simulink model "signal_builder"  (R2019b)
settings: Solver=VariableStepAuto  StartTime=0.0  StopTime=8760  RelTol=1e-3
undefined symbols (not defined in the file or in its folder): sigbuilder_block
settings Model: Creator=HP  LastModifiedBy=HP

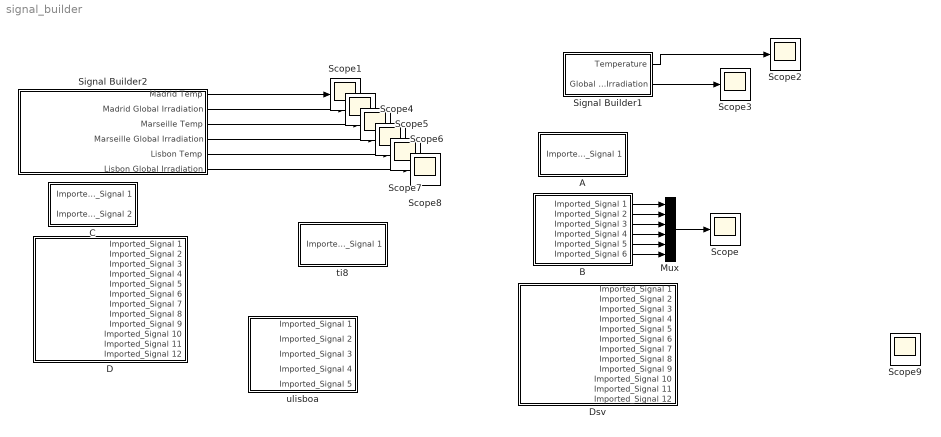
== system signal_builder ==
  A : Subsystem  Tag=STV Subsys  LoadFcn=sigbuilder_block('load');  StartFcn=sigbuilder_block('start');  StopFcn=sigbuilder_block('stop');  ClipboardFcn=sigbuilder_block('clipboard');  mask(Sigbuilder block){tuvar=[0:10]}
      mask help: Simulink:masks:SigbuilderBlock_MD
      mask init:
      | if ~strcmp(get_param(bdroot(gcbh),'SimulationStatus'),'stopped') tuvar = sigbuilder_block('maskInit'); end
      settings: CopyFcn=sigbuilder_block('copy');  DeleteFcn=sigbuilder_block('delete');  ModelCloseFcn=sigbuilder_block('modelClose');  PreSaveFcn=sigbuilder_block('preSave');  PauseFcn=sigbuilder_block('pause');  ContinueFcn=sigbuilder_block('continue');  NameChangeFcn=sigbuilder_block('namechange');  OpenFcn=sigbuilder_block('open',[437.6 153 550.4 359.25 ]);  CloseFcn=sigbuilder_block('close');
      mask Display: plot(0, 0, 100, 100,[2, 2, 32, 32, 2], [68, 8, 8, 68, 68],[32, 2], [38, 38], [32, 19, 2],[53, 60, 44], [32, 17, 17, 2],[16, 16, 31, 31]);txt = getActiveGroup(gcbh);text(2, 100, txt,'verticalAlignment', 'top');
  B : Subsystem  Tag=STV Subsys  LoadFcn=sigbuilder_block('load');  StartFcn=sigbuilder_block('start');  StopFcn=sigbuilder_block('stop');  ClipboardFcn=sigbuilder_block('clipboard');  mask(Sigbuilder block){tuvar=[0:10]}
      mask help: Simulink:masks:SigbuilderBlock_MD
      mask init:
      | if ~strcmp(get_param(bdroot(gcbh),'SimulationStatus'),'stopped') tuvar = sigbuilder_block('maskInit'); end
      settings: CopyFcn=sigbuilder_block('copy');  DeleteFcn=sigbuilder_block('delete');  ModelCloseFcn=sigbuilder_block('modelClose');  PreSaveFcn=sigbuilder_block('preSave');  PauseFcn=sigbuilder_block('pause');  ContinueFcn=sigbuilder_block('continue');  NameChangeFcn=sigbuilder_block('namechange');  OpenFcn=sigbuilder_block('open',[0 0 762.75 233.25 ]);  CloseFcn=sigbuilder_block('close');
      mask Display: plot(0, 0, 100, 100,[2, 2, 32, 32, 2], [68, 8, 8, 68, 68],[32, 2], [38, 38], [32, 19, 2],[53, 60, 44], [32, 17, 17, 2],[16, 16, 31, 31]);txt = getActiveGroup(gcbh);text(2, 100, txt,'verticalAlignment', 'top');
  C : Subsystem  Tag=STV Subsys  LoadFcn=sigbuilder_block('load');  StartFcn=sigbuilder_block('start');  StopFcn=sigbuilder_block('stop');  ClipboardFcn=sigbuilder_block('clipboard');  mask(Sigbuilder block){tuvar=[0:10]}
      mask help: Simulink:masks:SigbuilderBlock_MD
      mask init:
      | if ~strcmp(get_param(bdroot(gcbh),'SimulationStatus'),'stopped') tuvar = sigbuilder_block('maskInit'); end
      settings: CopyFcn=sigbuilder_block('copy');  DeleteFcn=sigbuilder_block('delete');  ModelCloseFcn=sigbuilder_block('modelClose');  PreSaveFcn=sigbuilder_block('preSave');  PauseFcn=sigbuilder_block('pause');  ContinueFcn=sigbuilder_block('continue');  NameChangeFcn=sigbuilder_block('namechange');  OpenFcn=sigbuilder_block('open',[440.25 156.75 544.5 355.5 ]);  CloseFcn=sigbuilder_block('close');
      mask Display: plot(0, 0, 100, 100,[2, 2, 32, 32, 2], [68, 8, 8, 68, 68],[32, 2], [38, 38], [32, 19, 2],[53, 60, 44], [32, 17, 17, 2],[16, 16, 31, 31]);txt = getActiveGroup(gcbh);text(2, 100, txt,'verticalAlignment', 'top');
  D : Subsystem  Tag=STV Subsys  LoadFcn=sigbuilder_block('load');  StartFcn=sigbuilder_block('start');  StopFcn=sigbuilder_block('stop');  ClipboardFcn=sigbuilder_block('clipboard');  mask(Sigbuilder block){tuvar=[0:10]}
      mask help: Simulink:masks:SigbuilderBlock_MD
      mask init:
      | if ~strcmp(get_param(bdroot(gcbh),'SimulationStatus'),'stopped') tuvar = sigbuilder_block('maskInit'); end
      settings: CopyFcn=sigbuilder_block('copy');  DeleteFcn=sigbuilder_block('delete');  ModelCloseFcn=sigbuilder_block('modelClose');  PreSaveFcn=sigbuilder_block('preSave');  PauseFcn=sigbuilder_block('pause');  ContinueFcn=sigbuilder_block('continue');  NameChangeFcn=sigbuilder_block('namechange');  OpenFcn=sigbuilder_block('open',[6 30 1012.5 447.75 ]);  CloseFcn=sigbuilder_block('close');
      mask Display: plot(0, 0, 100, 100,[2, 2, 32, 32, 2], [68, 8, 8, 68, 68],[32, 2], [38, 38], [32, 19, 2],[53, 60, 44], [32, 17, 17, 2],[16, 16, 31, 31]);txt = getActiveGroup(gcbh);text(2, 100, txt,'verticalAlignment', 'top');
  Dsv : Subsystem  Tag=STV Subsys  LoadFcn=sigbuilder_block('load');  StartFcn=sigbuilder_block('start');  StopFcn=sigbuilder_block('stop');  ClipboardFcn=sigbuilder_block('clipboard');  mask(Sigbuilder block){tuvar=[0:10]}
      mask help: Simulink:masks:SigbuilderBlock_MD
      mask init:
      | if ~strcmp(get_param(bdroot(gcbh),'SimulationStatus'),'stopped') tuvar = sigbuilder_block('maskInit'); end
      settings: CopyFcn=sigbuilder_block('copy');  DeleteFcn=sigbuilder_block('delete');  ModelCloseFcn=sigbuilder_block('modelClose');  PreSaveFcn=sigbuilder_block('preSave');  PauseFcn=sigbuilder_block('pause');  ContinueFcn=sigbuilder_block('continue');  NameChangeFcn=sigbuilder_block('namechange');  OpenFcn=sigbuilder_block('open',[361.5 30 657 447.75 ]);  CloseFcn=sigbuilder_block('close');
      mask Display: plot(0, 0, 100, 100,[2, 2, 32, 32, 2], [68, 8, 8, 68, 68],[32, 2], [38, 38], [32, 19, 2],[53, 60, 44], [32, 17, 17, 2],[16, 16, 31, 31]);txt = getActiveGroup(gcbh);text(2, 100, txt,'verticalAlignment', 'top');
  Mux : Mux  Inputs=6
  Scope{,1..9} (10 alike) : Scope
  Signal Builder1 : Subsystem  Tag=STV Subsys  LoadFcn=sigbuilder_block('load');  StartFcn=sigbuilder_block('start');  StopFcn=sigbuilder_block('stop');  ClipboardFcn=sigbuilder_block('clipboard');  mask(Sigbuilder block){tuvar=[0:10]}
      mask help: Simulink:masks:SigbuilderBlock_MD
      mask init:
      | if ~strcmp(get_param(bdroot(gcbh),'SimulationStatus'),'stopped') tuvar = sigbuilder_block('maskInit'); end
      settings: CopyFcn=sigbuilder_block('copy');  DeleteFcn=sigbuilder_block('delete');  ModelCloseFcn=sigbuilder_block('modelClose');  PreSaveFcn=sigbuilder_block('preSave');  PauseFcn=sigbuilder_block('pause');  ContinueFcn=sigbuilder_block('continue');  NameChangeFcn=sigbuilder_block('namechange');  OpenFcn=sigbuilder_block('open',[82.5 73.5 550.5 359.25 ]);  CloseFcn=sigbuilder_block('close');
      mask Display: plot(0, 0, 100, 100,[2, 2, 32, 32, 2], [68, 8, 8, 68, 68],[32, 2], [38, 38], [32, 19, 2],[53, 60, 44], [32, 17, 17, 2],[16, 16, 31, 31]);txt = getActiveGroup(gcbh);text(2, 100, txt,'verticalAlignment', 'top');
  Signal Builder2 : Subsystem  Tag=STV Subsys  LoadFcn=sigbuilder_block('load');  StartFcn=sigbuilder_block('start');  StopFcn=sigbuilder_block('stop');  ClipboardFcn=sigbuilder_block('clipboard');  mask(Sigbuilder block){tuvar=[0:10]}
      mask help: Simulink:masks:SigbuilderBlock_MD
      mask init:
      | if ~strcmp(get_param(bdroot(gcbh),'SimulationStatus'),'stopped') tuvar = sigbuilder_block('maskInit'); end
      settings: CopyFcn=sigbuilder_block('copy');  DeleteFcn=sigbuilder_block('delete');  ModelCloseFcn=sigbuilder_block('modelClose');  PreSaveFcn=sigbuilder_block('preSave');  PauseFcn=sigbuilder_block('pause');  ContinueFcn=sigbuilder_block('continue');  NameChangeFcn=sigbuilder_block('namechange');  OpenFcn=sigbuilder_block('open',[6 30 1012.5 447.75 ]);  CloseFcn=sigbuilder_block('close');
      mask Display: plot(0, 0, 100, 100,[2, 2, 32, 32, 2], [68, 8, 8, 68, 68],[32, 2], [38, 38], [32, 19, 2],[53, 60, 44], [32, 17, 17, 2],[16, 16, 31, 31]);txt = getActiveGroup(gcbh);text(2, 100, txt,'verticalAlignment', 'top');
  ti8 : Subsystem  Tag=STV Subsys  LoadFcn=sigbuilder_block('load');  StartFcn=sigbuilder_block('start');  StopFcn=sigbuilder_block('stop');  ClipboardFcn=sigbuilder_block('clipboard');  mask(Sigbuilder block){tuvar=[0:10]}
      mask help: Simulink:masks:SigbuilderBlock_MD
      mask init:
      | if ~strcmp(get_param(bdroot(gcbh),'SimulationStatus'),'stopped') tuvar = sigbuilder_block('maskInit'); end
      settings: CopyFcn=sigbuilder_block('copy');  DeleteFcn=sigbuilder_block('delete');  ModelCloseFcn=sigbuilder_block('modelClose');  PreSaveFcn=sigbuilder_block('preSave');  PauseFcn=sigbuilder_block('pause');  ContinueFcn=sigbuilder_block('continue');  NameChangeFcn=sigbuilder_block('namechange');  OpenFcn=sigbuilder_block('open',[437.6 153 550.4 359.25 ]);  CloseFcn=sigbuilder_block('close');
      mask Display: plot(0, 0, 100, 100,[2, 2, 32, 32, 2], [68, 8, 8, 68, 68],[32, 2], [38, 38], [32, 19, 2],[53, 60, 44], [32, 17, 17, 2],[16, 16, 31, 31]);txt = getActiveGroup(gcbh);text(2, 100, txt,'verticalAlignment', 'top');
  ulisboa : Subsystem  Tag=STV Subsys  LoadFcn=sigbuilder_block('load');  StartFcn=sigbuilder_block('start');  StopFcn=sigbuilder_block('stop');  ClipboardFcn=sigbuilder_block('clipboard');  mask(Sigbuilder block){tuvar=[0:10]}
      mask help: Simulink:masks:SigbuilderBlock_MD
      mask init:
      | if ~strcmp(get_param(bdroot(gcbh),'SimulationStatus'),'stopped') tuvar = sigbuilder_block('maskInit'); end
      settings: CopyFcn=sigbuilder_block('copy');  DeleteFcn=sigbuilder_block('delete');  ModelCloseFcn=sigbuilder_block('modelClose');  PreSaveFcn=sigbuilder_block('preSave');  PauseFcn=sigbuilder_block('pause');  ContinueFcn=sigbuilder_block('continue');  NameChangeFcn=sigbuilder_block('namechange');  OpenFcn=sigbuilder_block('open',[437.6 153 550.4 359.25 ]);  CloseFcn=sigbuilder_block('close');
      mask Display: plot(0, 0, 100, 100,[2, 2, 32, 32, 2], [68, 8, 8, 68, 68],[32, 2], [38, 38], [32, 19, 2],[53, 60, 44], [32, 17, 17, 2],[16, 16, 31, 31]);txt = getActiveGroup(gcbh);text(2, 100, txt,'verticalAlignment', 'top');
  wires:
  Signal Builder1/1(Temperature) -> Scope2/1
  Signal Builder1/2(Global Irradiation) -> Scope3/1
  Signal Builder2/1(Madrid Temp) -> Scope1/1
  Signal Builder2/2(Madrid Global Irradiation) -> Scope4/1
  Signal Builder2/3(Marseille Temp) -> Scope5/1
  Signal Builder2/4(Marseille Global Irradiation) -> Scope6/1
  Signal Builder2/5(Lisbon Temp) -> Scope7/1
  Signal Builder2/6(Lisbon Global Irradiation) -> Scope8/1
  B/2(Imported_Signal 2) -> Mux/2
  B/3(Imported_Signal 3) -> Mux/3
  B/4(Imported_Signal 4) -> Mux/4
  B/6(Imported_Signal 6) -> Mux/6
  B/1(Imported_Signal 1) -> Mux/1
  B/5(Imported_Signal 5) -> Mux/5
  Mux/1 -> Scope/1

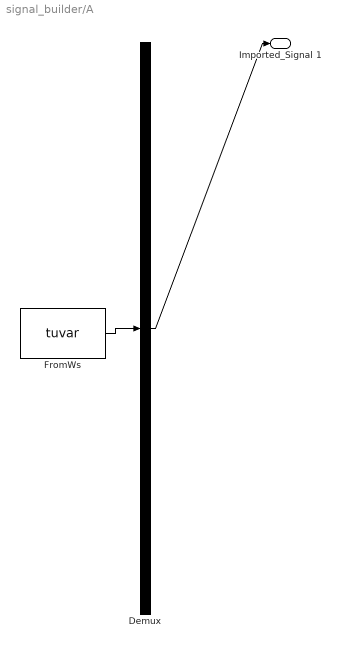
== system signal_builder/A ==
  Demux : Demux  Tag=STV Demux  Outputs=1
  FromWs : FromWorkspace  Tag=STV FromWs  VariableName=tuvar  SampleTime=0
      SigBuilderData=|
      | common.afterFinalStr = 'Extrapolate'
      | common.sampleTime = 0
      | dataSet.timeRange = [0 9000]
      | dataSet.name = 'Group 1'
      | sbobj.Groups.Name = 'Group 1'
      | sbobj.Groups.Signals.Name = 'Imported_Signal 1'
      | sbobj.Groups.Signals.XData = [0 2 3 4 5 6 7 8 9 10 11 12 ... (8760 elements, 1x8760)]
      | sbobj.Groups.Signals.YData = [-0.0152836915327 -0.0152836915327 -0.0152836915327 -0.0152836915327 -0.0152836915327 -0.0204334354339 -0.0204334354339 -0.00970029681324 -0.00970029681324 -0.00970029681324 -0.00970029681324 -0.00970029681324 ... (8760 elements, 1x8760)]
      | sbobj.Groups.TimeRange = [0 9000]
  Imported_Signal 1 : Outport  Tag=STV Outport
  wires:
  FromWs/1 -> Demux/1
  Demux/1 -> Imported_Signal 1/1

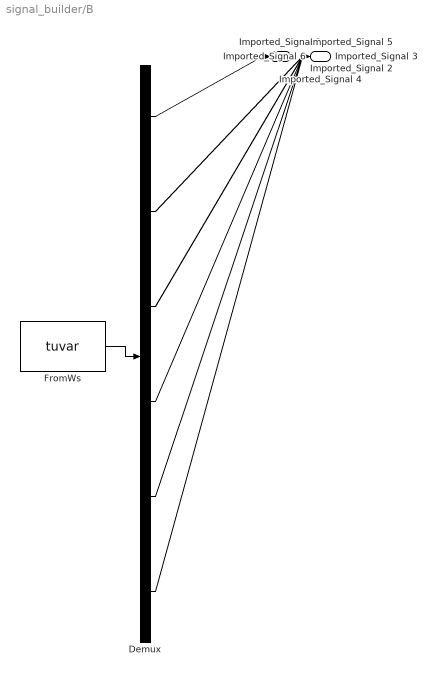
== system signal_builder/B ==
  Demux : Demux  Tag=STV Demux  Outputs=6
  FromWs : FromWorkspace  Tag=STV FromWs  VariableName=tuvar  SampleTime=0
      SigBuilderData=|
      | common.afterFinalStr = 'Extrapolate'
      | common.sampleTime = 0
      | dataSet.timeRange = [0 9000]
      | dataSet.name = 'Group 1'
      | sbobj.Groups.Name = 'Group 1'
      | sbobj.Groups.Signals(1).Name = 'Imported_Signal 1'
      | sbobj.Groups.Signals(1).XData = [0 2 3 4 5 6 7 8 9 10 11 12 ... (8760 elements, 1x8760)]
      | sbobj.Groups.Signals(1).YData = [0.00967357699951 0.00967357699951 0.00967357699951 0.00967357699951 0.00967357699951 0.00964893245892 0.00964893245892 0.00970029681324 0.00970029681324 0.00970029681324 0.00970029681324 0.00970029681324 ... (8760 elements, 1x8760)]
      | sbobj.Groups.Signals(2).Name = 'Imported_Signal 2'
      | sbobj.Groups.Signals(2).XData = [0 2 3 4 5 6 7 8 9 10 11 12 ... (8760 elements, 1x8760)]
      | sbobj.Groups.Signals(2).YData = [0.00561011453317 0.00561011453317 0.00561011453317 0.00561011453317 0.00561011453317 0.0107845029749 0.0107845029749 0 0 0 0 0 ... (8760 elements, 1x8760)]
      | sbobj.Groups.Signals(3).Name = 'Imported_Signal 3'
      | sbobj.Groups.Signals(3).XData = [0 2 3 4 5 6 7 8 9 10 11 12 ... (8760 elements, 1x8760)]
      | sbobj.Groups.Signals(3).YData = [9578966887.67 9578966887.67 9578966887.67 9578966887.67 9578966887.67 9578966887.67 9578966887.67 9578966887.67 9578966887.67 9578966887.67 9578966887.67 9578966887.67 ... (8760 elements, 1x8760)]
      | sbobj.Groups.Signals(4).Name = 'Imported_Signal 4'
      | sbobj.Groups.Signals(4).XData = [0 2 3 4 5 6 7 8 9 10 11 12 ... (8760 elements, 1x8760)]
      | sbobj.Groups.Signals(4).YData = [9393082762.66 9393082762.66 9393082762.66 9393082762.66 9393082762.66 9263715095.51 9263715095.51 9533344252.07 9533344252.07 9533344252.07 9533344252.07 9533344252.07 ... (8760 elements, 1x8760)]
      | sbobj.Groups.Signals(5).Name = 'Imported_Signal 5'
      | sbobj.Groups.Signals(5).XData = [0 2 3 4 5 6 7 8 9 10 11 12 ... (8760 elements, 1x8760)]
      | sbobj.Groups.Signals(5).YData = [9147423011.85 9147423011.85 9147423011.85 9147423011.85 9147423011.85 8791475482.96 8791475482.96 9533344252.07 9533344252.07 9533344252.07 9533344252.07 9533344252.07 ... (8760 elements, 1x8760)]
      | sbobj.Groups.Signals(6).Name = 'Imported_Signal 6'
      | sbobj.Groups.Signals(6).XData = [0 2 3 4 5 6 7 8 9 10 11 12 ... (8760 elements, 1x8760)]
      | sbobj.Groups.Signals(6).YData = [9147423011.85 9147423011.85 9147423011.85 9147423011.85 9147423011.85 8791475482.96 8791475482.96 9533344252.07 9533344252.07 9533344252.07 9533344252.07 9533344252.07 ... (8760 elements, 1x8760)]
      | sbobj.Groups.TimeRange = [0 9000]
  Imported_Signal 1 : Outport  Tag=STV Outport
  Imported_Signal 2 : Outport  Tag=STV Outport  Port=2
  Imported_Signal 3 : Outport  Tag=STV Outport  Port=3
  Imported_Signal 4 : Outport  Tag=STV Outport  Port=4
  Imported_Signal 5 : Outport  Tag=STV Outport  Port=5
  Imported_Signal 6 : Outport  Tag=STV Outport  Port=6
  wires:
  FromWs/1 -> Demux/1
  Demux/1 -> Imported_Signal 1/1
  Demux/2 -> Imported_Signal 2/1
  Demux/3 -> Imported_Signal 3/1
  Demux/4 -> Imported_Signal 4/1
  Demux/5 -> Imported_Signal 5/1
  Demux/6 -> Imported_Signal 6/1

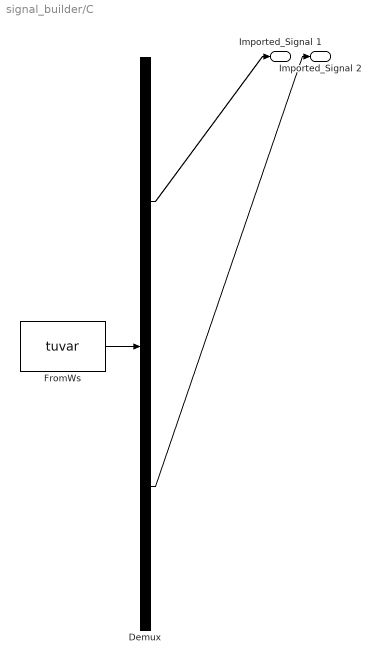
== system signal_builder/C ==
  Demux : Demux  Tag=STV Demux  Outputs=2
  FromWs : FromWorkspace  Tag=STV FromWs  VariableName=tuvar  SampleTime=0
      SigBuilderData=|
      | common.afterFinalStr = 'Extrapolate'
      | common.sampleTime = 0
      | dataSet.timeRange = [0 9000]
      | dataSet.name = 'Group 1'
      | sbobj.Groups.Name = 'Group 1'
      | sbobj.Groups.Signals(1).Name = 'Imported_Signal 1'
      | sbobj.Groups.Signals(1).XData = [0 2 3 4 5 6 7 8 9 10 11 12 ... (8760 elements, 1x8760)]
      | sbobj.Groups.Signals(1).YData = [0.954948808062 0.954948808062 0.954948808062 0.954948808062 0.954948808062 0.917789526371 0.917789526371 0.995237207088 0.995237207088 0.995237207088 0.995237207088 0.995237207088 ... (8760 elements, 1x8760)]
      | sbobj.Groups.Signals(2).Name = 'Imported_Signal 2'
      | sbobj.Groups.Signals(2).XData = [0 2 3 4 5 6 7 8 9 10 11 12 ... (8760 elements, 1x8760)]
      | sbobj.Groups.Signals(2).YData = [0.980594553965 0.980594553965 0.980594553965 0.980594553965 0.980594553965 0.967089165684 0.967089165684 0.995237207088 0.995237207088 0.995237207088 0.995237207088 0.995237207088 ... (8760 elements, 1x8760)]
      | sbobj.Groups.TimeRange = [0 9000]
  Imported_Signal 1 : Outport  Tag=STV Outport
  Imported_Signal 2 : Outport  Tag=STV Outport  Port=2
  wires:
  FromWs/1 -> Demux/1
  Demux/1 -> Imported_Signal 1/1
  Demux/2 -> Imported_Signal 2/1

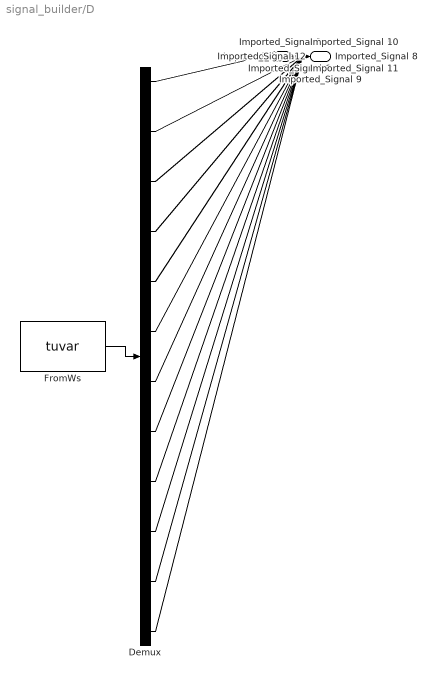
== system signal_builder/D ==
  Demux : Demux  Tag=STV Demux  Outputs=12
  FromWs : FromWorkspace  Tag=STV FromWs  VariableName=tuvar  SampleTime=0
      SigBuilderData=|
      | common.afterFinalStr = 'Extrapolate'
      | common.sampleTime = 0
      | dataSet.timeRange = [0 9000]
      | dataSet.name = 'Group 1'
      | sbobj.Groups.Name = 'Group 1'
      | sbobj.Groups.Signals(1).Name = 'Imported_Signal 1'
      | sbobj.Groups.Signals(1).XData = [0 2 3 4 5 6 7 8 9 10 11 12 ... (8760 elements, 1x8760)]
      | sbobj.Groups.Signals(1).YData = [0.00456998932691 0.00456998932691 0.00456998932691 0.00456998932691 0.00456998932691 0.00439216040112 0.00439216040112 0.00476279291176 0.00476279291176 0.00476279291176 0.00476279291176 0.00476279291176 ... (8760 elements, 1x8760)]
      | sbobj.Groups.Signals(2).Name = 'Imported_Signal 2'
      | sbobj.Groups.Signals(2).XData = [0 2 3 4 5 6 7 8 9 10 11 12 ... (8760 elements, 1x8760)]
      | sbobj.Groups.Signals(2).YData = [0.0404812026106 0.0404812026106 0.0404812026106 0.0404812026106 0.0404812026106 0.0778183132275 0.0778183132275 0 0 0 0 0 ... (8760 elements, 1x8760)]
      | sbobj.Groups.Signals(3).Name = 'Imported_Signal 3'
      | sbobj.Groups.Signals(3).XData = [0 2 3 4 5 6 7 8 9 10 11 12 ... (8760 elements, 1x8760)]
      | sbobj.Groups.Signals(3).YData = [0 0 0 0 0 0 0 0 0 0 0 0 ... (8760 elements, 1x8760)]
      | sbobj.Groups.Signals(4).Name = 'Imported_Signal 4'
      | sbobj.Groups.Signals(4).XData = [0 2 3 4 5 6 7 8 9 10 11 12 ... (8760 elements, 1x8760)]
      | sbobj.Groups.Signals(4).YData = [0.000239894452856 0.000239894452856 0.000239894452856 0.000239894452856 0.000239894452856 0.000230559601109 0.000230559601109 0.000250015375946 0.000250015375946 0.000250015375946 0.000250015375946 0.000250015375946 ... (8760 elements, 1x8760)]
      | sbobj.Groups.Signals(5).Name = 'Imported_Signal 5'
      | sbobj.Groups.Signals(5).XData = [0 2 3 4 5 6 7 8 9 10 11 12 ... (8760 elements, 1x8760)]
      | sbobj.Groups.Signals(5).YData = [0.000660055480363 0.000660055480363 0.000660055480363 0.000660055480363 0.000660055480363 0.000634371184703 0.000634371184703 0.000687902605096 0.000687902605096 0.000687902605096 0.000687902605096 0.000687902605096 ... (8760 elements, 1x8760)]
      | sbobj.Groups.Signals(6).Name = 'Imported_Signal 6'
      | sbobj.Groups.Signals(6).XData = [0 2 3 4 5 6 7 8 9 10 11 12 ... (8760 elements, 1x8760)]
      | sbobj.Groups.Signals(6).YData = [0.000660055480363 0.000660055480363 0.000660055480363 0.000660055480363 0.000660055480363 0.000634371184703 0.000634371184703 0.000687902605096 0.000687902605096 0.000687902605096 0.000687902605096 0.000687902605096 ... (8760 elements, 1x8760)]
      | sbobj.Groups.Signals(7).Name = 'Imported_Signal 7'
      | sbobj.Groups.Signals(7).XData = [0 2 3 4 5 6 7 8 9 10 11 12 ... (8760 elements, 1x8760)]
      | sbobj.Groups.Signals(7).YData = [0.00469271924088 0.00469271924088 0.00469271924088 0.00469271924088 0.00469271924088 0.00462808804831 0.00462808804831 0.00476279291176 0.00476279291176 0.00476279291176 0.00476279291176 0.00476279291176 ... (8760 elements, 1x8760)]
      | sbobj.Groups.Signals(8).Name = 'Imported_Signal 8'
      | sbobj.Groups.Signals(8).XData = [0 2 3 4 5 6 7 8 9 10 11 12 ... (8760 elements, 1x8760)]
      | sbobj.Groups.Signals(8).YData = [0.0147127267937 0.0147127267937 0.0147127267937 0.0147127267937 0.0147127267937 0.028282746268 0.028282746268 0 0 0 0 0 ... (8760 elements, 1x8760)]
      | sbobj.Groups.Signals(9).Name = 'Imported_Signal 9'
      | sbobj.Groups.Signals(9).XData = [0 2 3 4 5 6 7 8 9 10 11 12 ... (8760 elements, 1x8760)]
      | sbobj.Groups.Signals(9).YData = [0 0 0 0 0 0 0 0 0 0 0 0 ... (8760 elements, 1x8760)]
      | sbobj.Groups.Signals(10).Name = 'Imported_Signal 10'
      | sbobj.Groups.Signals(10).XData = [0 2 3 4 5 6 7 8 9 10 11 12 ... (8760 elements, 1x8760)]
      | sbobj.Groups.Signals(10).YData = [0.000246336968025 0.000246336968025 0.000246336968025 0.000246336968025 0.000246336968025 0.000242944254505 0.000242944254505 0.000250015375946 0.000250015375946 0.000250015375946 0.000250015375946 0.000250015375946 ... (8760 elements, 1x8760)]
      | sbobj.Groups.Signals(11).Name = 'Imported_Signal 11'
      | sbobj.Groups.Signals(11).XData = [0 2 3 4 5 6 7 8 9 10 11 12 ... (8760 elements, 1x8760)]
      | sbobj.Groups.Signals(11).YData = [0.000239894452856 0.000239894452856 0.000239894452856 0.000239894452856 0.000239894452856 0.000230559601109 0.000230559601109 0.000250015375946 0.000250015375946 0.000250015375946 0.000250015375946 0.000250015375946 ... (8760 elements, 1x8760)]
      | sbobj.Groups.Signals(12).Name = 'Imported_Signal 12'
      | sbobj.Groups.Signals(12).XData = [0 2 3 4 5 6 7 8 9 10 11 12 ... (8760 elements, 1x8760)]
      | sbobj.Groups.Signals(12).YData = [0.000239894452856 0.000239894452856 0.000239894452856 0.000239894452856 0.000239894452856 0.000230559601109 0.000230559601109 0.000250015375946 0.000250015375946 0.000250015375946 0.000250015375946 0.000250015375946 ... (8760 elements, 1x8760)]
      | sbobj.Groups.TimeRange = [0 9000]
  Imported_Signal 1 : Outport  Tag=STV Outport
  Imported_Signal 2 : Outport  Tag=STV Outport  Port=2
  Imported_Signal 3 : Outport  Tag=STV Outport  Port=3
  Imported_Signal 4 : Outport  Tag=STV Outport  Port=4
  Imported_Signal 5 : Outport  Tag=STV Outport  Port=5
  Imported_Signal 6 : Outport  Tag=STV Outport  Port=6
  Imported_Signal 7 : Outport  Tag=STV Outport  Port=7
  Imported_Signal 8 : Outport  Tag=STV Outport  Port=8
  Imported_Signal 9 : Outport  Tag=STV Outport  Port=9
  Imported_Signal 10 : Outport  Tag=STV Outport  Port=10
  Imported_Signal 11 : Outport  Tag=STV Outport  Port=11
  Imported_Signal 12 : Outport  Tag=STV Outport  Port=12
  wires:
  FromWs/1 -> Demux/1
  Demux/1 -> Imported_Signal 1/1
  Demux/2 -> Imported_Signal 2/1
  Demux/3 -> Imported_Signal 3/1
  Demux/4 -> Imported_Signal 4/1
  Demux/5 -> Imported_Signal 5/1
  Demux/6 -> Imported_Signal 6/1
  Demux/7 -> Imported_Signal 7/1
  Demux/8 -> Imported_Signal 8/1
  Demux/9 -> Imported_Signal 9/1
  Demux/10 -> Imported_Signal 10/1
  Demux/11 -> Imported_Signal 11/1
  Demux/12 -> Imported_Signal 12/1

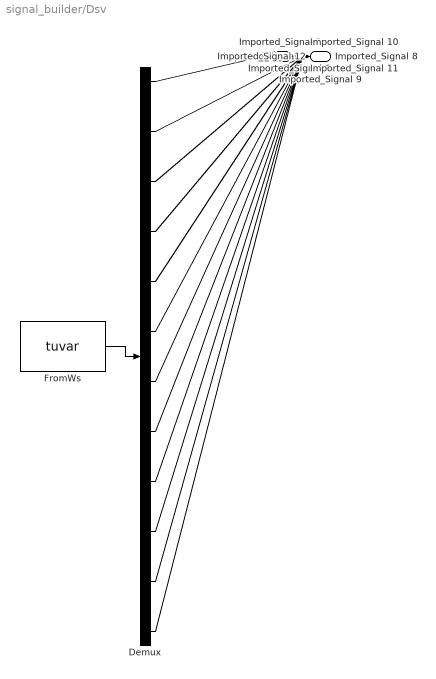
== system signal_builder/Dsv ==
  Demux : Demux  Tag=STV Demux  Outputs=12
  FromWs : FromWorkspace  Tag=STV FromWs  VariableName=tuvar  SampleTime=0
      SigBuilderData=|
      | common.afterFinalStr = 'Extrapolate'
      | common.sampleTime = 0
      | dataSet.timeRange = [0 9000]
      | dataSet.name = 'Group 1'
      | sbobj.Groups.Name = 'Group 1'
      | sbobj.Groups.Signals(1).Name = 'Imported_Signal 1'
      | sbobj.Groups.Signals(1).XData = [0 2 3 4 5 6 7 8 9 10 11 12 ... (8760 elements, 1x8760)]
      | sbobj.Groups.Signals(1).YData = [0.00456998932691 0.00456998932691 0.00456998932691 0.00456998932691 0.00456998932691 0.00439216040112 0.00439216040112 0.00476279291176 0.00476279291176 0.00476279291176 0.00476279291176 0.00476279291176 ... (8760 elements, 1x8760)]
      | sbobj.Groups.Signals(2).Name = 'Imported_Signal 2'
      | sbobj.Groups.Signals(2).XData = [0 2 3 4 5 6 7 8 9 10 11 12 ... (8760 elements, 1x8760)]
      | sbobj.Groups.Signals(2).YData = [0.00469271924088 0.00469271924088 0.00469271924088 0.00469271924088 0.00469271924088 0.00462808804831 0.00462808804831 0.00476279291176 0.00476279291176 0.00476279291176 0.00476279291176 0.00476279291176 ... (8760 elements, 1x8760)]
      | sbobj.Groups.Signals(3).Name = 'Imported_Signal 3'
      | sbobj.Groups.Signals(3).XData = [0 2 3 4 5 6 7 8 9 10 11 12 ... (8760 elements, 1x8760)]
      | sbobj.Groups.Signals(3).YData = [0.0404812026106 0.0404812026106 0.0404812026106 0.0404812026106 0.0404812026106 0.0778183132275 0.0778183132275 0 0 0 0 0 ... (8760 elements, 1x8760)]
      | sbobj.Groups.Signals(4).Name = 'Imported_Signal 4'
      | sbobj.Groups.Signals(4).XData = [0 2 3 4 5 6 7 8 9 10 11 12 ... (8760 elements, 1x8760)]
      | sbobj.Groups.Signals(4).YData = [0.0147127267937 0.0147127267937 0.0147127267937 0.0147127267937 0.0147127267937 0.028282746268 0.028282746268 0 0 0 0 0 ... (8760 elements, 1x8760)]
      | sbobj.Groups.Signals(5).Name = 'Imported_Signal 5'
      | sbobj.Groups.Signals(5).XData = [0 2 3 4 5 6 7 8 9 10 11 12 ... (8760 elements, 1x8760)]
      | sbobj.Groups.Signals(5).YData = [0 0 0 0 0 0 0 0 0 0 0 0 ... (8760 elements, 1x8760)]
      | sbobj.Groups.Signals(6).Name = 'Imported_Signal 6'
      | sbobj.Groups.Signals(6).XData = [0 2 3 4 5 6 7 8 9 10 11 12 ... (8760 elements, 1x8760)]
      | sbobj.Groups.Signals(6).YData = [0 0 0 0 0 0 0 0 0 0 0 0 ... (8760 elements, 1x8760)]
      | sbobj.Groups.Signals(7).Name = 'Imported_Signal 7'
      | sbobj.Groups.Signals(7).XData = [0 2 3 4 5 6 7 8 9 10 11 12 ... (8760 elements, 1x8760)]
      | sbobj.Groups.Signals(7).YData = [0.000239894452856 0.000239894452856 0.000239894452856 0.000239894452856 0.000239894452856 0.000230559601109 0.000230559601109 0.000250015375946 0.000250015375946 0.000250015375946 0.000250015375946 0.000250015375946 ... (8760 elements, 1x8760)]
      | sbobj.Groups.Signals(8).Name = 'Imported_Signal 8'
      | sbobj.Groups.Signals(8).XData = [0 2 3 4 5 6 7 8 9 10 11 12 ... (8760 elements, 1x8760)]
      | sbobj.Groups.Signals(8).YData = [0.000246336968025 0.000246336968025 0.000246336968025 0.000246336968025 0.000246336968025 0.000242944254505 0.000242944254505 0.000250015375946 0.000250015375946 0.000250015375946 0.000250015375946 0.000250015375946 ... (8760 elements, 1x8760)]
      | sbobj.Groups.Signals(9).Name = 'Imported_Signal 9'
      | sbobj.Groups.Signals(9).XData = [0 2 3 4 5 6 7 8 9 10 11 12 ... (8760 elements, 1x8760)]
      | sbobj.Groups.Signals(9).YData = [0.000660055480363 0.000660055480363 0.000660055480363 0.000660055480363 0.000660055480363 0.000634371184703 0.000634371184703 0.000687902605096 0.000687902605096 0.000687902605096 0.000687902605096 0.000687902605096 ... (8760 elements, 1x8760)]
      | sbobj.Groups.Signals(10).Name = 'Imported_Signal 10'
      | sbobj.Groups.Signals(10).XData = [0 2 3 4 5 6 7 8 9 10 11 12 ... (8760 elements, 1x8760)]
      | sbobj.Groups.Signals(10).YData = [0.000239894452856 0.000239894452856 0.000239894452856 0.000239894452856 0.000239894452856 0.000230559601109 0.000230559601109 0.000250015375946 0.000250015375946 0.000250015375946 0.000250015375946 0.000250015375946 ... (8760 elements, 1x8760)]
      | sbobj.Groups.Signals(11).Name = 'Imported_Signal 11'
      | sbobj.Groups.Signals(11).XData = [0 2 3 4 5 6 7 8 9 10 11 12 ... (8760 elements, 1x8760)]
      | sbobj.Groups.Signals(11).YData = [0.000660055480363 0.000660055480363 0.000660055480363 0.000660055480363 0.000660055480363 0.000634371184703 0.000634371184703 0.000687902605096 0.000687902605096 0.000687902605096 0.000687902605096 0.000687902605096 ... (8760 elements, 1x8760)]
      | sbobj.Groups.Signals(12).Name = 'Imported_Signal 12'
      | sbobj.Groups.Signals(12).XData = [0 2 3 4 5 6 7 8 9 10 11 12 ... (8760 elements, 1x8760)]
      | sbobj.Groups.Signals(12).YData = [0.000239894452856 0.000239894452856 0.000239894452856 0.000239894452856 0.000239894452856 0.000230559601109 0.000230559601109 0.000250015375946 0.000250015375946 0.000250015375946 0.000250015375946 0.000250015375946 ... (8760 elements, 1x8760)]
      | sbobj.Groups.TimeRange = [0 9000]
  Imported_Signal 1 : Outport  Tag=STV Outport
  Imported_Signal 2 : Outport  Tag=STV Outport  Port=2
  Imported_Signal 3 : Outport  Tag=STV Outport  Port=3
  Imported_Signal 4 : Outport  Tag=STV Outport  Port=4
  Imported_Signal 5 : Outport  Tag=STV Outport  Port=5
  Imported_Signal 6 : Outport  Tag=STV Outport  Port=6
  Imported_Signal 7 : Outport  Tag=STV Outport  Port=7
  Imported_Signal 8 : Outport  Tag=STV Outport  Port=8
  Imported_Signal 9 : Outport  Tag=STV Outport  Port=9
  Imported_Signal 10 : Outport  Tag=STV Outport  Port=10
  Imported_Signal 11 : Outport  Tag=STV Outport  Port=11
  Imported_Signal 12 : Outport  Tag=STV Outport  Port=12
  wires:
  FromWs/1 -> Demux/1
  Demux/1 -> Imported_Signal 1/1
  Demux/2 -> Imported_Signal 2/1
  Demux/3 -> Imported_Signal 3/1
  Demux/4 -> Imported_Signal 4/1
  Demux/5 -> Imported_Signal 5/1
  Demux/6 -> Imported_Signal 6/1
  Demux/7 -> Imported_Signal 7/1
  Demux/8 -> Imported_Signal 8/1
  Demux/9 -> Imported_Signal 9/1
  Demux/10 -> Imported_Signal 10/1
  Demux/11 -> Imported_Signal 11/1
  Demux/12 -> Imported_Signal 12/1

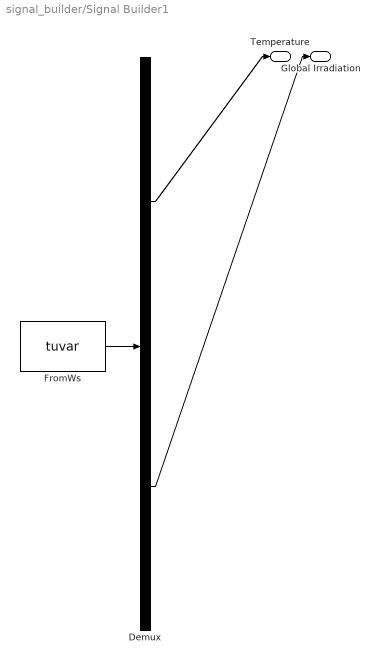
== system signal_builder/Signal Builder1 ==
  Demux : Demux  Tag=STV Demux  Outputs=2
  FromWs : FromWorkspace  Tag=STV FromWs  VariableName=tuvar  SampleTime=0
      SigBuilderData=|
      | common.afterFinalStr = 'Extrapolate'
      | common.sampleTime = 0
      | dataSet.timeRange = [0 9000]
      | dataSet.name = 'Group 1'
      | sbobj.Groups.Name = 'Group 1'
      | sbobj.Groups.Signals(1).Name = 'Temperature'
      | sbobj.Groups.Signals(1).XData = [0 1 2 3 4 5 6 7 8 9 10 11 ... (8761 elements, 1x8761)]
      | sbobj.Groups.Signals(1).YData = [10.5 10.4 10.4 10.3 10.2 10.1 10 10.2 10.7 11.6 12.6 13.8 ... (8761 elements, 1x8761)]
      | sbobj.Groups.Signals(2).Name = 'Global Irradiation'
      | sbobj.Groups.Signals(2).XData = [0 1 2 3 4 5 6 7 8 9 10 11 ... (8760 elements, 1x8760)]
      | sbobj.Groups.Signals(2).YData = [0 0 0 0 0 0 0 0 55.5 180 298 381 ... (8760 elements, 1x8760)]
      | sbobj.Groups.TimeRange = [0 9000]
  Temperature : Outport  Tag=STV Outport
  Global Irradiation : Outport  Tag=STV Outport  Port=2
  wires:
  FromWs/1 -> Demux/1
  Demux/1 -> Temperature/1
  Demux/2 -> Global Irradiation/1

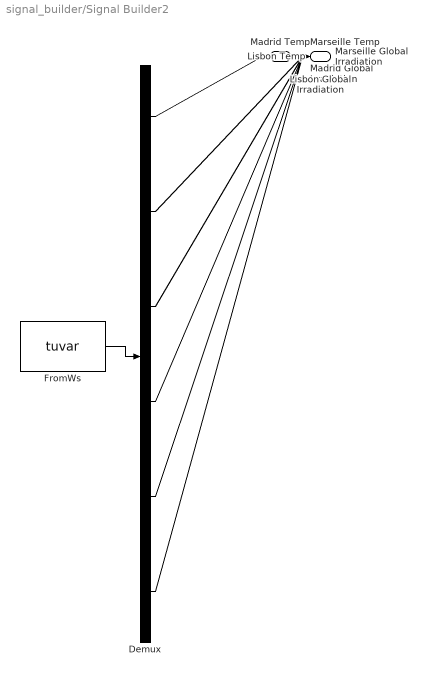
== system signal_builder/Signal Builder2 ==
  Demux : Demux  Tag=STV Demux  Outputs=6
  FromWs : FromWorkspace  Tag=STV FromWs  VariableName=tuvar  SampleTime=0
      SigBuilderData=|
      | common.afterFinalStr = 'Extrapolate'
      | common.sampleTime = 0
      | dataSet.timeRange = [0 9000]
      | dataSet.name = 'Group 1'
      | sbobj.Groups.Name = 'Group 1'
      | sbobj.Groups.Signals(1).Name = 'Madrid Temp'
      | sbobj.Groups.Signals(1).XData = [0 1 2 3 4 5 6 7 8 9 10 11 ... (8760 elements, 1x8760)]
      | sbobj.Groups.Signals(1).YData = [9.7 9.7 9.5 9.2 8.8 8.3 7 7.3 7.7 8 9.3 10.7 ... (8760 elements, 1x8760)]
      | sbobj.Groups.Signals(2).Name = 'Madrid Global Irradiation'
      | sbobj.Groups.Signals(2).XData = [0 1 2 3 4 5 6 7 8 9 10 11 ... (8760 elements, 1x8760)]
      | sbobj.Groups.Signals(2).YData = [0 0 0 0 0 0 0 0 1.2 12 125.492590491 349.631721109 ... (8760 elements, 1x8760)]
      | sbobj.Groups.Signals(3).Name = 'Marseille Temp'
      | sbobj.Groups.Signals(3).XData = [0 1 2 3 4 5 6 7 8 9 10 11 ... (8761 elements, 1x8761)]
      | sbobj.Groups.Signals(3).YData = [9.4 8.9 8.6 8.4 8.3 8.1 6.9 5 6 6.3 7 9 ... (8761 elements, 1x8761)]
      | sbobj.Groups.Signals(4).Name = 'Marseille Global Irradiation'
      | sbobj.Groups.Signals(4).XData = [0 1 2 3 4 5 6 7 8 9 10 11 ... (8760 elements, 1x8760)]
      | sbobj.Groups.Signals(4).YData = [0 0 0 0 0 0 0 0 4.2 32.4 242.750743786 444.341360946 ... (8760 elements, 1x8760)]
      | sbobj.Groups.Signals(5).Name = 'Lisbon Temp'
      | sbobj.Groups.Signals(5).XData = [0 1 2 3 4 5 6 7 8 9 10 11 ... (8761 elements, 1x8761)]
      | sbobj.Groups.Signals(5).YData = [10.5 10.4 10.4 10.3 10.2 10.1 10 10.2 10.7 11.6 12.6 13.8 ... (8761 elements, 1x8761)]
      | sbobj.Groups.Signals(6).Name = 'Lisbon Global Irradiation'
      | sbobj.Groups.Signals(6).XData = [0 1 2 3 4 5 6 7 8 9 10 11 ... (8760 elements, 1x8760)]
      | sbobj.Groups.Signals(6).YData = [0 0 0 0 0 0 0 0 55.5 180 298 381 ... (8760 elements, 1x8760)]
      | sbobj.Groups.TimeRange = [0 9000]
  Madrid Temp : Outport  Tag=STV Outport
  Madrid Global Irradiation : Outport  Tag=STV Outport  Port=2
  Marseille Temp : Outport  Tag=STV Outport  Port=3
  Marseille Global Irradiation : Outport  Tag=STV Outport  Port=4
  Lisbon Temp : Outport  Tag=STV Outport  Port=5
  Lisbon Global Irradiation : Outport  Tag=STV Outport  Port=6
  wires:
  FromWs/1 -> Demux/1
  Demux/1 -> Madrid Temp/1
  Demux/2 -> Madrid Global Irradiation/1
  Demux/3 -> Marseille Temp/1
  Demux/4 -> Marseille Global Irradiation/1
  Demux/5 -> Lisbon Temp/1
  Demux/6 -> Lisbon Global Irradiation/1

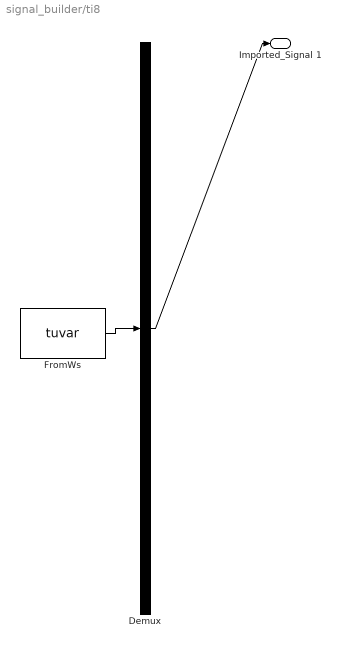
== system signal_builder/ti8 ==
  Demux : Demux  Tag=STV Demux  Outputs=1
  FromWs : FromWorkspace  Tag=STV FromWs  VariableName=tuvar  SampleTime=0
      SigBuilderData=|
      | common.afterFinalStr = 'Extrapolate'
      | common.sampleTime = 0
      | dataSet.timeRange = [0 9000]
      | dataSet.name = 'Group 1'
      | sbobj.Groups.Name = 'Group 1'
      | sbobj.Groups.Signals.Name = 'Imported_Signal 1'
      | sbobj.Groups.Signals.XData = [0 1 2 3 4 5 6 7 8 9 10 11 ... (8762 elements, 1x8762)]
      | sbobj.Groups.Signals.YData = [87.4271110737 28.4140666123 19.7272309787 20.3511071141 20.1171937327 20.2012169219 20.2457456789 20.2112182185 20.0628700021 20.1238779764 20.1427206093 20.1146153596 ... (8762 elements, 1x8762)]
      | sbobj.Groups.TimeRange = [0 9000]
  Imported_Signal 1 : Outport  Tag=STV Outport
  wires:
  FromWs/1 -> Demux/1
  Demux/1 -> Imported_Signal 1/1

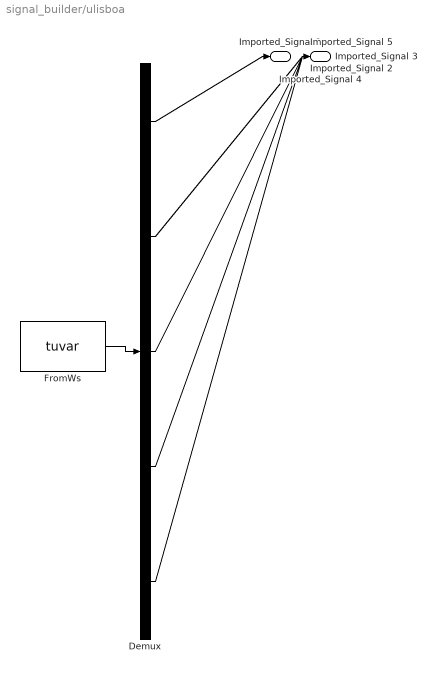
== system signal_builder/ulisboa ==
  Demux : Demux  Tag=STV Demux  Outputs=5
  FromWs : FromWorkspace  Tag=STV FromWs  VariableName=tuvar  SampleTime=0
      SigBuilderData=|
      | common.afterFinalStr = 'Extrapolate'
      | common.sampleTime = 0
      | dataSet.timeRange = [0 9000]
      | dataSet.name = 'Group 1'
      | sbobj.Groups.Name = 'Group 1'
      | sbobj.Groups.Signals(1).Name = 'Imported_Signal 1'
      | sbobj.Groups.Signals(1).XData = [0 1 2 3 4 5 6 7 8 9 10 11 ... (8762 elements, 1x8762)]
      | sbobj.Groups.Signals(1).YData = [10.3 10.3 10.5 10.4 10.4 10.3 10.2 10.1 10 10.2 10.7 11.6 ... (8762 elements, 1x8762)]
      | sbobj.Groups.Signals(2).Name = 'Imported_Signal 2'
      | sbobj.Groups.Signals(2).XData = [0 1 2 3 4 5 6 7 8 9 10 11 ... (8762 elements, 1x8762)]
      | sbobj.Groups.Signals(2).YData = [10.3 10.3 10.5 10.4 10.4 10.3 10.2 10.1 20 20 20 20 ... (8762 elements, 1x8762)]
      | sbobj.Groups.Signals(3).Name = 'Imported_Signal 3'
      | sbobj.Groups.Signals(3).XData = [0 1 2 3 4 5 6 7 8 9 10 11 ... (8762 elements, 1x8762)]
      | sbobj.Groups.Signals(3).YData = [63.3950307067 63.3950307067 75.2897198881 75.0094543369 75.5336603617 75.2533948105 240.708683745 240.427180397 2000 2000 2000 2000 ... (8762 elements, 1x8762)]
      | sbobj.Groups.Signals(4).Name = 'Imported_Signal 4'
      | sbobj.Groups.Signals(4).XData = [0 1 2 3 4 5 6 7 8 9 10 11 ... (8762 elements, 1x8762)]
      | sbobj.Groups.Signals(4).YData = [32.2317868014 32.2317868014 38.2793757289 38.1368809719 38.4034018119 38.2609070549 122.382951616 122.239827529 -12.0329759534 -17.2014646062 281.045007622 409.965673888 ... (8762 elements, 1x8762)]
      | sbobj.Groups.Signals(5).Name = 'Imported_Signal 5'
      | sbobj.Groups.Signals(5).XData = [0 2 3 4 5 6 7 8 9 10 11 12 ... (8760 elements, 1x8760)]
      | sbobj.Groups.Signals(5).YData = [150 150 150 150 150 400 400 0 0 0 0 0 ... (8760 elements, 1x8760)]
      | sbobj.Groups.TimeRange = [0 9000]
  Imported_Signal 1 : Outport  Tag=STV Outport
  Imported_Signal 2 : Outport  Tag=STV Outport  Port=2
  Imported_Signal 3 : Outport  Tag=STV Outport  Port=3
  Imported_Signal 4 : Outport  Tag=STV Outport  Port=4
  Imported_Signal 5 : Outport  Tag=STV Outport  Port=5
  wires:
  FromWs/1 -> Demux/1
  Demux/1 -> Imported_Signal 1/1
  Demux/2 -> Imported_Signal 2/1
  Demux/3 -> Imported_Signal 3/1
  Demux/4 -> Imported_Signal 4/1
  Demux/5 -> Imported_Signal 5/1
